simulink model "Series_and_Parallel"  (R2024b)
settings: Solver=VariableStepAuto  StartTime=0.0  StopTime=10.0  RelTol=1e-3
libraries: spsSeriesRLCBranchLib x11, spsVoltageMeasurementLib x11, spsCurrentMeasurementLib x8, spsACVoltageSourceLib x2, spsDCVoltageSourceLib x2, sps_lib x1
settings Model: Creator=priya  LastModifiedBy=priya

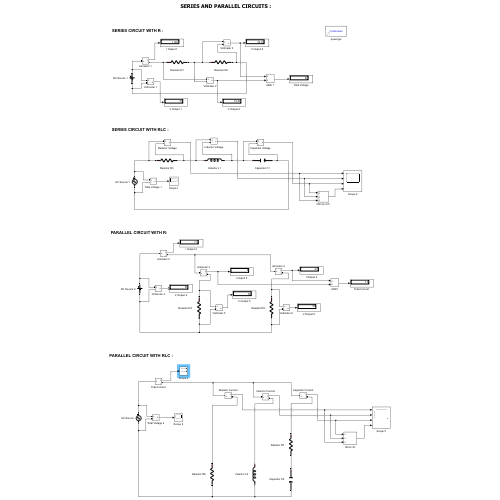
[thumbnail: Simulink's stored preview of the top-level diagram]
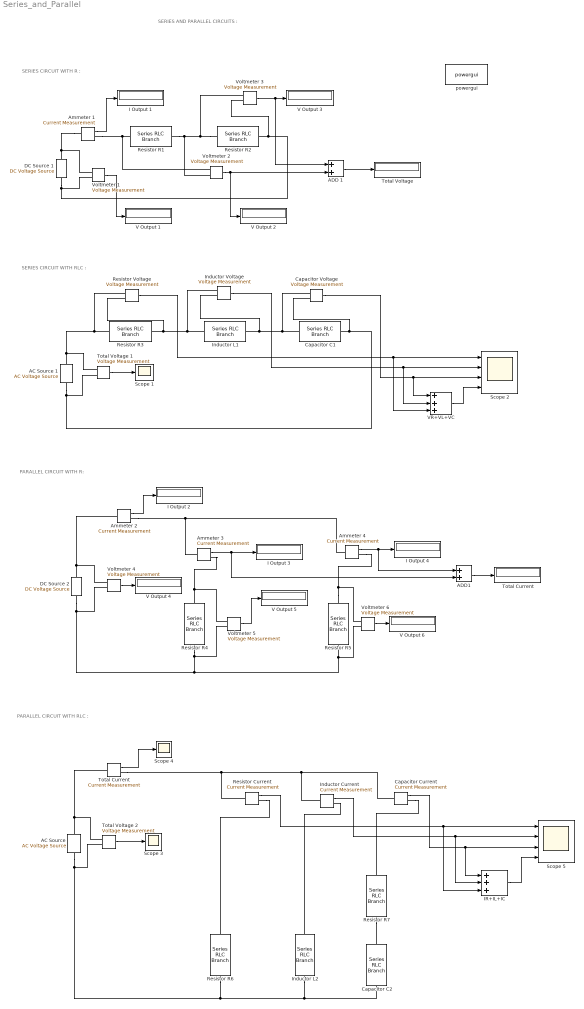
== system Series_and_Parallel ==
  note: SERIES CIRCUIT WITH RLC :
  note: PARALLEL CIRCUIT WITH R:
  note: SERIES CIRCUIT WITH R :
  note: SERIES AND PARALLEL CIRCUITS :
  note: PARALLEL CIRCUIT WITH RLC :
  AC Source : spsACVoltageSourceLib/AC Voltage Source  Amplitude=50  Phase=0  Frequency=60  SampleTime=0  Measurements=None  BusType=swing  Pref=10e3  Qref=0  Qmin=-inf  Qmax=+inf
  AC Source 1 : spsACVoltageSourceLib/AC Voltage Source  Amplitude=50  Phase=0  Frequency=60  SampleTime=0  Measurements=None  BusType=swing  Pref=10e3  Qref=0  Qmin=-inf  Qmax=+inf
  ADD 1 : Sum
  ADD1 : Sum
  Ammeter {1..4} (4 alike) : spsCurrentMeasurementLib/Current Measurement  PhasorSimulation=off  OutputType=Complex  PSBequivalent=0
  Capacitor C1 : spsSeriesRLCBranchLib/Series RLC Branch  LConnTagsString=__new0  RConnTagsString=__new0  BranchType=C  Resistance=10  Inductance=1e-3  SetiL0=off  InitialCurrent=0  Capacitance=7.04e-4  Setx0=off  InitialVoltage=0  Measurements=None
  Capacitor C2 : spsSeriesRLCBranchLib/Series RLC Branch  LConnTagsString=__new0  RConnTagsString=__new0  BranchType=C  Resistance=10  Inductance=1e-3  SetiL0=off  InitialCurrent=0  Capacitance=7.04e-4  Setx0=off  InitialVoltage=0  Measurements=None
  Capacitor Current : spsCurrentMeasurementLib/Current Measurement  PhasorSimulation=off  OutputType=Complex  PSBequivalent=0
  Capacitor Voltage : spsVoltageMeasurementLib/Voltage Measurement  PhasorSimulation=off  OutputType=Complex  PSBequivalent=0
  DC Source 1 : spsDCVoltageSourceLib/DC Voltage Source  Amplitude=50  Measurements=None
  DC Source 2 : spsDCVoltageSourceLib/DC Voltage Source  Amplitude=50  Measurements=None
  I Output {1..4} (4 alike) : Display
  IR+IL+IC : Sum  Inputs=+++
  Inductor Current : spsCurrentMeasurementLib/Current Measurement  PhasorSimulation=off  OutputType=Complex  PSBequivalent=0
  Inductor L1 : spsSeriesRLCBranchLib/Series RLC Branch  LConnTagsString=__new0  RConnTagsString=__new0  BranchType=L  Resistance=10  Inductance=0.01  SetiL0=off  InitialCurrent=0  Capacitance=1e-6  Setx0=off  InitialVoltage=0  Measurements=None
  Inductor L2 : spsSeriesRLCBranchLib/Series RLC Branch  LConnTagsString=__new0  RConnTagsString=__new0  BranchType=L  Resistance=10  Inductance=0.01  SetiL0=off  InitialCurrent=0  Capacitance=1e-6  Setx0=off  InitialVoltage=0  Measurements=None
  Inductor Voltage : spsVoltageMeasurementLib/Voltage Measurement  PhasorSimulation=off  OutputType=Complex  PSBequivalent=0
  Resistor Current : spsCurrentMeasurementLib/Current Measurement  PhasorSimulation=off  OutputType=Complex  PSBequivalent=0
  Resistor R1 : spsSeriesRLCBranchLib/Series RLC Branch  LConnTagsString=__new0  RConnTagsString=__new0  BranchType=R  Resistance=10  Inductance=1e-3  SetiL0=off  InitialCurrent=0  Capacitance=1e-6  Setx0=off  InitialVoltage=0  Measurements=None
  Resistor R2 : spsSeriesRLCBranchLib/Series RLC Branch  LConnTagsString=__new0  RConnTagsString=__new0  BranchType=R  Resistance=20  Inductance=1e-3  SetiL0=off  InitialCurrent=0  Capacitance=1e-6  Setx0=off  InitialVoltage=0  Measurements=None
  Resistor R3 : spsSeriesRLCBranchLib/Series RLC Branch  LConnTagsString=__new0  RConnTagsString=__new0  BranchType=R  Resistance=10  Inductance=1e-3  SetiL0=off  InitialCurrent=0  Capacitance=1e-6  Setx0=off  InitialVoltage=0  Measurements=None
  "Resistor R4 " : spsSeriesRLCBranchLib/Series RLC Branch  LConnTagsString=__new0  RConnTagsString=__new0  BranchType=R  Resistance=10  Inductance=1e-3  SetiL0=off  InitialCurrent=0  Capacitance=1e-6  Setx0=off  InitialVoltage=0  Measurements=None
  Resistor R5 : spsSeriesRLCBranchLib/Series RLC Branch  LConnTagsString=__new0  RConnTagsString=__new0  BranchType=R  Resistance=20  Inductance=1e-3  SetiL0=off  InitialCurrent=0  Capacitance=1e-6  Setx0=off  InitialVoltage=0  Measurements=None
  Resistor R6 : spsSeriesRLCBranchLib/Series RLC Branch  LConnTagsString=__new0  RConnTagsString=__new0  BranchType=R  Resistance=10  Inductance=1e-3  SetiL0=off  InitialCurrent=0  Capacitance=1e-6  Setx0=off  InitialVoltage=0  Measurements=None
  Resistor R7 : spsSeriesRLCBranchLib/Series RLC Branch  LConnTagsString=__new0  RConnTagsString=__new0  BranchType=R  Resistance=1e-3  Inductance=1e-3  SetiL0=off  InitialCurrent=0  Capacitance=1e-6  Setx0=off  InitialVoltage=0  Measurements=None
  Resistor Voltage : spsVoltageMeasurementLib/Voltage Measurement  PhasorSimulation=off  OutputType=Complex  PSBequivalent=0
  Scope 1 : Scope
  Scope 2 : Scope  NumInputPorts=4
  Scope 3 : Scope
  Scope 4 : Scope
  Scope 5 : Scope  NumInputPorts=4
  Total Current : spsCurrentMeasurementLib/Current Measurement  PhasorSimulation=off  OutputType=Complex  PSBequivalent=0
  "Total Current " : Display
  Total Voltage : Display
  Total Voltage 1 : spsVoltageMeasurementLib/Voltage Measurement  PhasorSimulation=off  OutputType=Complex  PSBequivalent=0
  Total Voltage 2 : spsVoltageMeasurementLib/Voltage Measurement  PhasorSimulation=off  OutputType=Complex  PSBequivalent=0
  V Output {1..6} (6 alike) : Display
  VR+VL+VC : Sum  Inputs=+++
  Voltmeter {1..6} (6 alike) : spsVoltageMeasurementLib/Voltage Measurement  PhasorSimulation=off  OutputType=Complex  PSBequivalent=0
  powergui : sps_lib/powergui  Priority=1  SimulationMode=Continuous  SampleTime=1e-6  frequency=60  Iterations=50  frequencyindice=0  Pbase=100e6  ErrMax=1e-4  UnitsV=kV  UnitsW=MW  buscounter=0  FunctionMessages=off  echomessages=off  EnableUseOfTLC=off  CurrentSourceSwitches=off  DisableSnubberDevices=off  DisableRonSwitches=off  DisableVfSwitches=off  DisplayEquations=off  AutomaticDiscreteSolvers=off  SolverType=Tustin/Backward Euler (TBE)  Interpol=off  ExternalGateDelay=off  methode=off  Ts=100  x0status=blocks  SPID=on  SwTol=0  HookPort=off  NonlinearTolerance=1e-4  nMaxIteration=100  ContinueOnMaxIteration=off  RestoreLinks=warning  ResistiveCurrentMeasurement=off  Frange=[0:2:500]  Ylog=off  Xlog=on  ShowGrid=off  save=off  variable=ZData  structure=0  ZoomFFT=off  StartTime=0.0  cycles=1  DisplayStyle=1  fundamental=60  FreqAxis=off  MaxFrequency=1000  frequencyindicesteady=1  RmsSteady=1  display=off
  wires:
  Voltmeter 6/1 -> V Output 6/1
  Ammeter 1/1 -> I Output 1/1
  Ammeter 4/1 -> ADD1/1, I Output 4/1
  Voltmeter 2/1 -> V Output 2/1, ADD 1/2
  Voltmeter 5/1 -> V Output 5/1
  Voltmeter 3/1 -> ADD 1/1, V Output 3/1
  Ammeter 2/1 -> I Output 2/1
  Voltmeter 4/1 -> V Output 4/1
  Voltmeter 1/1 -> V Output 1/1
  ADD 1/1 -> Total Voltage/1
  Ammeter 3/1 -> ADD1/2, I Output 3/1
  Resistor Voltage/1 -> VR+VL+VC/3, Scope 2/1
  Inductor Voltage/1 -> VR+VL+VC/2, Scope 2/2
  Resistor Current/1 -> Scope 5/1, IR+IL+IC/3
  Inductor Current/1 -> Scope 5/2, IR+IL+IC/2
  Capacitor Current/1 -> Scope 5/3, IR+IL+IC/1
  Total Voltage 1/1 -> Scope 1/1
  Capacitor Voltage/1 -> VR+VL+VC/1, Scope 2/3
  ADD1/1 -> "Total Current "/1
  Total Voltage 2/1 -> Scope 3/1
  Total Current/1 -> Scope 4/1
  VR+VL+VC/1 -> Scope 2/4
  IR+IL+IC/1 -> Scope 5/4
  connections:
  Resistor R2/RConn1 -- DC Source 1/LConn1 -- Voltmeter 1/LConn2 -- Voltmeter 3/LConn2
  Ammeter 4/LConn1 -- Ammeter 2/RConn1 -- Ammeter 3/LConn1
  Ammeter 3/RConn1 -- Voltmeter 5/LConn1 -- "Resistor R4 "/LConn1
  Resistor R5/RConn1 -- Voltmeter 4/LConn2 -- DC Source 2/LConn1 -- Voltmeter 5/LConn2 -- "Resistor R4 "/RConn1 -- Voltmeter 6/LConn2
  Resistor R5/LConn1 -- Ammeter 4/RConn1 -- Voltmeter 6/LConn1
  Voltmeter 4/LConn1 -- DC Source 2/RConn1 -- Ammeter 2/LConn1
  Resistor R2/LConn1 -- Voltmeter 3/LConn1 -- Resistor R1/RConn1 -- Voltmeter 2/LConn2
  Resistor R1/LConn1 -- Ammeter 1/RConn1 -- Voltmeter 2/LConn1
  Ammeter 1/LConn1 -- DC Source 1/RConn1 -- Voltmeter 1/LConn1
  Inductor L1/LConn1 -- Inductor Voltage/LConn1 -- Resistor Voltage/LConn2 -- Resistor R3/RConn1
  Capacitor C1/LConn1 -- Capacitor Voltage/LConn1 -- Inductor Voltage/LConn2 -- Inductor L1/RConn1
  AC Source 1/LConn1 -- Total Voltage 1/LConn2 -- Capacitor Voltage/LConn2 -- Capacitor C1/RConn1
  AC Source 1/RConn1 -- Resistor Voltage/LConn1 -- Resistor R3/LConn1 -- Total Voltage 1/LConn1
  Total Current/LConn1 -- AC Source/RConn1 -- Total Voltage 2/LConn1
  Total Voltage 2/LConn2 -- AC Source/LConn1 -- Capacitor C2/RConn1 -- Inductor L2/RConn1 -- Resistor R6/RConn1
  Resistor Current/LConn1 -- Inductor Current/LConn1 -- Capacitor Current/LConn1 -- Total Current/RConn1
  Resistor Current/RConn1 -- Resistor R6/LConn1
  Inductor Current/RConn1 -- Inductor L2/LConn1
  Resistor R7/RConn1 -- Capacitor C2/LConn1
  Capacitor Current/RConn1 -- Resistor R7/LConn1
